simulink model "Q1_B1"  (R2020b)
settings: Solver=ode45  StartTime=0.0  StopTime=100  RelTol=1e-3  EnableMultiTasking=on
libraries: pid_lib x1
settings Model: Creator=SENAI LAPTOP  LastModifiedBy=RISHIKESH_SREEKUMAR
settings DataIOCC: LimitDataPoints=on  SaveFormat=Array  ReturnWorkspaceOutputs=off
settings OptimizationCC: LifeSpan=inf
settings DebuggingCC: SolverPrmCheckMsg=warning  SFUnexpectedBacktrackingDiag=warning  SFNoUnconditionalDefaultTransitionDiag=warning  SFExecutionAtInitializationDiag=none  ArithmeticOperatorsInVariantConditions=warning
settings HardwareCC: ProdBitPerPointer=32  ProdBitPerSizeT=32  ProdBitPerPtrDiffT=32  ProdLargestAtomicFloat=None  ProdIntDivRoundTo=Undefined  ProdEndianess=Unspecified  ProdWordSize=32  ProdHWDeviceType=32-bit Generic
settings ModelReferenceCC: PropagateSignalLabelsOutOfModel=off
settings SFSimCC: SimUseLocalCustomCode=off  CustomCodeUndefinedFunction=UseInterfaceOnly
settings RTWCC: RTWUseLocalCustomCode=off
settings CodeAppCC: StateflowObjectComments=on
settings GRTTargetCC: TargetLangStandard=C89/C90 (ANSI)
settings ConfigComp: CovMetricSettings=dw  CovSaveCumulativeToWorkspaceVar=on  CovSaveSingleToWorkspaceVar=on  CovExternalEMLEnable=off  CovSFcnEnable=off

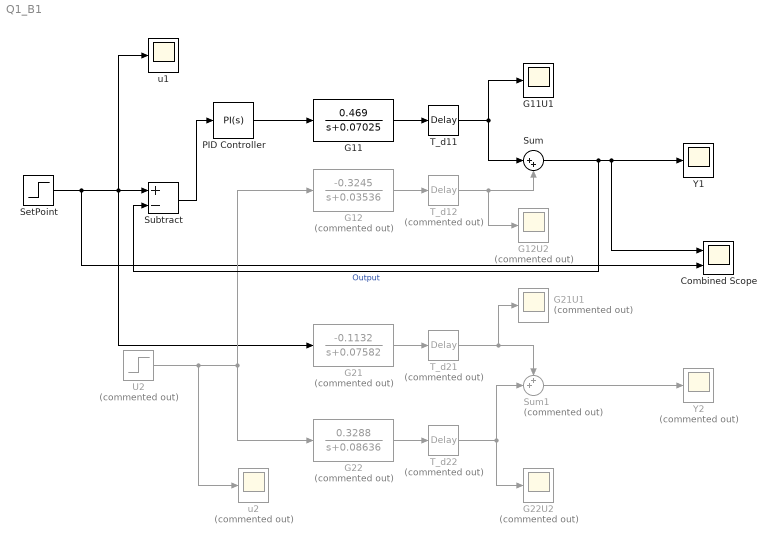
== system Q1_B1 ==
  Combined Scope : Scope  NumInputPorts=2
  G11 : TransferFcn  Numerator=[0.469]  Denominator=[1 0.07025]
  G11U1 : Scope
  G12 : TransferFcn  Commented=on  Numerator=[-0.3245]  Denominator=[1 0.03536]
  G12U2 : Scope  Commented=on
  G21 : TransferFcn  Commented=on  Numerator=[-0.1132]  Denominator=[1 0.07582]
  G21U1 : Scope  Commented=on
  G22 : TransferFcn  Commented=on  Numerator=[0.3288]  Denominator=[1 0.08636]
  G22U2 : Scope  Commented=on
  PID Controller : pid_lib/PID Controller  Controller=PI  Form=Parallel  TimeDomain=Continuous-time  UseExternalTs=off  SampleTime=-1  IntegratorMethod=Forward Euler  FilterMethod=Forward Euler  ControllerParametersSource=internal  P=0.22952  I=0.02531  D=0.1366  UseFilter=on  N=0.2153  TunerSelectOption=Transfer Function Based (PID Tuner App)  InitialConditionSource=internal  InitialConditionForIntegrator=0  InitialConditionForFilter=0  DifferentiatorICPrevScaledInput=0  ExternalReset=none  TrackingMode=off  Kt=1  LimitOutput=off  SatLimitsSource=internal  UpperSaturationLimit=inf  LowerSaturationLimit=-inf  LinearizeAsGain=on  AntiWindupMode=none  Kb=1  POutMin=[]  POutMax=[]  IOutMin=[]  IOutMax=[]  DOutMin=[]  DOutMax=[]  NOutMin=[]  NOutMax=[]  SumOutMin=[]  SumOutMax=[]  SaturationOutMin=[]  SaturationOutMax=[]  PParamMin=[]  PParamMax=[]  IParamMin=[]  IParamMax=[]  DParamMin=[]  DParamMax=[]  NParamMin=[]  NParamMax=[]  KbParamMin=[]  KbParamMax=[]  KtParamMin=[]  KtParamMax=[]  KbOutMin=[]  KbOutMax=[]  KtOutMin=[]  KtOutMax=[]  IntegratorOutMin=[]  IntegratorOutMax=[]  FilterOutMin=[]  FilterOutMax=[]  SumI1OutMin=[]  SumI1OutMax=[]  SumI2OutMin=[]  SumI2OutMax=[]  SumI3OutMin=[]  SumI3OutMax=[]  SumI4OutMin=[]  SumI4OutMax=[]  SumDOutMin=[]  SumDOutMax=[]  DifferentiatorOutMin=[]  DifferentiatorOutMax=[]  FilterDiffOutCoefMin=[]  FilterDiffOutCoefMax=[]  ReciprocalOutMin=[]  ReciprocalOutMax=[]  SumDenOutMin=[]  SumDenOutMax=[]  SumNumOutMin=[]  SumNumOutMax=[]  DivideOutMin=[]  DivideOutMax=[]  UdiffTsProdOutMin=[]  UdiffTsProdOutMax=[]  NTsProdOutMin=[]  NTsProdOutMax=[]  UintegralTsProdOutMin=[]  UintegralTsProdOutMax=[]  UngainTsProdOutMin=[]  UngainTsProdOutMax=[]  IntegratorContinuousStateAttributes=''  IntegratorStateMustResolveToSignalObject=off  IntegratorRTWStateStorageClass=Auto  FilterContinuousStateAttributes=''  FilterStateMustResolveToSignalObject=off  FilterRTWStateStorageClass=Auto  ParallelPVariant=InternalParameters  IdealPVariant=Disabled  IVariant=InternalParameters  DVariant=Disabled  IntegratorVariant=Continuous  SatVariant=Disabled  AWVariant=Passthrough  PCopyVariant=Disabled  TRVariant=Disabled  FdbkBlocksVariant=Forward  IdealPFdbkVariant=Disabled  SatFdbkVariant=Disabled  DerivativeFilterVariant=Disabled  NVariant=Disabled  NCopyVariant=Disabled_SignalSpec  FilterICVariant=Disabled  IntegratorICVariant=InternalICs  ExternalResetVariant=Disabled  TRSumVariant=Passthrough  SumFdbkVariant=Disabled  SumVariant=Sum_PI  TsampFilterVariant=InternalTs  TsampNgainVariant=Passthrough  TsampIntegralVariant=Passthrough  ExternalSaturationOutDataTypeStr=Inherit: Same as second input
  SetPoint : Step  Time=10  SampleTime=0.1
  Subtract : Sum  Inputs=+-
  Sum : Sum  Inputs=|++
  Sum1 : Sum  Commented=on  Inputs=++|
  T_d11 : TransportDelay  DelayTime=2.5  PadeOrder=5
  T_d12 : TransportDelay  Commented=on  DelayTime=1.1  PadeOrder=5
  T_d21 : TransportDelay  Commented=on  DelayTime=1.1  PadeOrder=5
  "T_d22 " : TransportDelay  Commented=on  DelayTime=1.1  PadeOrder=5
  U2 : Step  Commented=on  Time=160  After=10  SampleTime=0.1
  Y1 : Scope
  Y2 : Scope  Commented=on
  u1 : Scope
  u2 : Scope  Commented=on
  wires:
  SetPoint/1 -> Combined Scope/2, u1/1, Subtract/1, G21/1
  G11/1 -> T_d11/1
  Sum1/1 -> Y2/1
  T_d11/1 -> G11U1/1, Sum/1
  T_d12/1 -> G12U2/1, Sum/2
  G12/1 -> T_d12/1
  T_d21/1 -> G21U1/1, Sum1/1
  G21/1 -> T_d21/1
  G22/1 -> "T_d22 "/1
  "T_d22 "/1 -> G22U2/1, Sum1/2
  U2/1 -> u2/1, G12/1, G22/1
  PID Controller/1 -> G11/1
  Subtract/1 -> PID Controller/1
  Sum/1 -> Subtract/2, Combined Scope/1, Y1/1  "Output"
